simulink model "vblast_MMSE"  (Simulink 7.6)
settings: Solver=ode45  StartTime=0.0  StopTime=10.0  RelTol=1e-3
libraries: commchan3 x12, commdigbbndpm3 x2, dspindex x2, commrandsrc2 x1, commsink2 x1, dspinverses x1
settings Model: Creator=Administrator  LastModifiedBy=Administrator

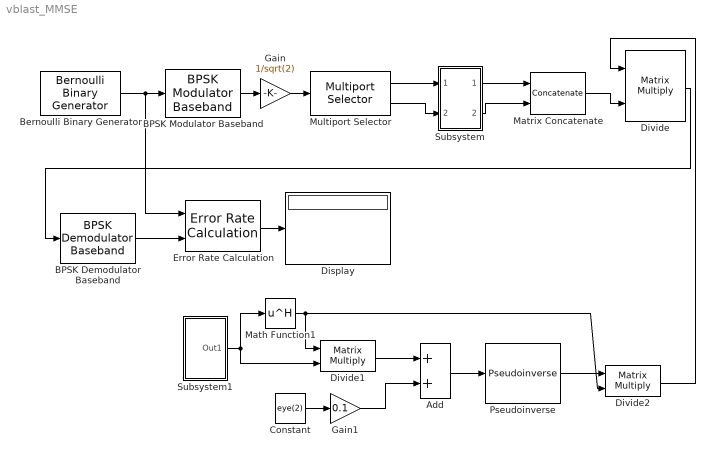
== system vblast_MMSE ==
  Add : Sum
  BPSK Demodulator Baseband : commdigbbndpm3/BPSK Demodulator Baseband  DialogController=commDDGCreate  DialogControllerArgs=DataTag0  Ph=0  DecType=Hard decision  VarSource=Dialog  Variance=1  outDtype=Inherit via internal rule  derotateFactorWordLen=16
  BPSK Modulator Baseband : commdigbbndpm3/BPSK Modulator Baseband  DialogController=commDDGCreate  DialogControllerArgs=DataTag1  SystemSampleTime=-1  Ph=0  outDtype=double  outWordLen=16  outUDDataType=sfix(16)  outFracLenMode=Best precision  outFracLen=15
  Bernoulli Binary Generator : commrandsrc2/Bernoulli Binary Generator  DialogController=commDDGCreate  DialogControllerArgs=DataTag2  SystemSampleTime=-1  P=0.5  seed=61  Ts=1e-6  frameBased=on  sampPerFrame=2  orient=off  outDataType=double
  Constant : Constant  Value=eye(2)
  Display : Display
  Divide : Product  Inputs=**  Multiplication=Matrix(*)
  Divide1 : Product  Inputs=**  Multiplication=Matrix(*)
  Divide2 : Product  Inputs=**  Multiplication=Matrix(*)
  Error Rate Calculation : commsink2/Error Rate Calculation  N=0  st_delay=0  cp_mode=Entire frame  subframe=[]  PMode=Port  WsName=ErrorVec  RsMode2=off  stop=off  numErr=100  maxBits=1e6
  Gain : Gain  Gain=1/sqrt(2)
  Gain1 : Gain  Gain=0.1
  Math Function1 : Math  Operator=hermitian  SaturateOnIntegerOverflow=on
  Matrix Concatenate : Concatenate  Mode=Multidimensional array
  Multiport Selector : dspindex/Multiport Selector  rowsOrCols=Rows  idxCellArray={ 1,2 }  idxErrMode=Clip Index
  Pseudoinverse : dspinverses/Pseudoinverse  wanterr=off
  Subsystem : Subsystem
  Subsystem1 : Subsystem
  wires:
  Bernoulli Binary Generator/1 -> BPSK Modulator Baseband/1, Error Rate Calculation/1
  BPSK Modulator Baseband/1 -> Gain/1
  Gain/1 -> Multiport Selector/1
  Subsystem/1(Out1) -> Matrix Concatenate/1
  Subsystem/2(Out2) -> Matrix Concatenate/2
  Multiport Selector/1 -> Subsystem/1(In1)
  Multiport Selector/2 -> Subsystem/2(In2)
  BPSK Demodulator Baseband/1 -> Error Rate Calculation/2
  Error Rate Calculation/1 -> Display/1
  Matrix Concatenate/1 -> Divide/2
  Divide/1 -> BPSK Demodulator Baseband/1
  Subsystem1/1(Out1) -> Math Function1/1, Divide1/2
  Math Function1/1 -> Divide1/1, Divide2/2
  Constant/1 -> Gain1/1
  Divide1/1 -> Add/1
  Gain1/1 -> Add/2
  Add/1 -> Pseudoinverse/1
  Pseudoinverse/1 -> Divide2/1
  Divide2/1 -> Divide/1

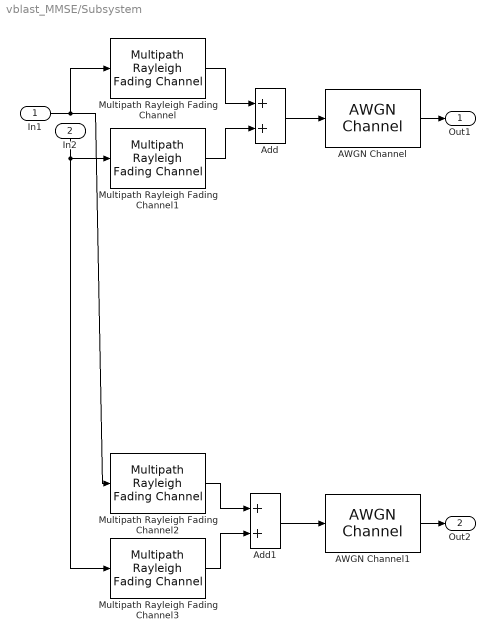
== system vblast_MMSE/Subsystem ==
  In1 : Inport
  In2 : Inport  Port=2
  AWGN Channel : commchan3/AWGN Channel  SystemSampleTime=-1  InputProcessing=Columns as channels (frame based)  seed=67  noiseMode="Signal to noise ratio  (SNR)"  EbNodB=10  EsNodB=10  SNRdB=10  bitsPerSym=1  Ps=1  Tsym=1  variance=1
  AWGN Channel1 : commchan3/AWGN Channel  SystemSampleTime=-1  InputProcessing=Columns as channels (frame based)  seed=671  noiseMode="Signal to noise ratio  (SNR)"  EbNodB=10  EsNodB=10  SNRdB=10  bitsPerSym=1  Ps=1  Tsym=1  variance=1
  Add : Sum
  Add1 : Sum
  Multipath Rayleigh Fading Channel : commchan3/Multipath Rayleigh Fading Channel  SystemSampleTime=-1  maxDopplerShift=40  spectrumType=Jakes  sigmaGaussian=1/sqrt(2)  coeffRounded=[1 -1.72 0.785]  freqMinMaxRJakes=[0 1]  freqMinMaxAJakes=[0 1]  sigmaGaussian1=1/sqrt(2)  sigmaGaussian2=1/sqrt(2)  centerFreqGaussian1=0.0  centerFreqGaussian2=0.0  gainGaussian1=0.5  gainGaussian2=0.5  coeffBell=9  dopplerSpectrum=doppler.jakes  pathDelays=0  avgPathGaindB=0  normalizePathGains=on  seed=73  enableProbe=0  openVisAtStart=off  outPathGains=off  outDelay=off
  Multipath Rayleigh Fading Channel1 : commchan3/Multipath Rayleigh Fading Channel  SystemSampleTime=-1  maxDopplerShift=40  spectrumType=Jakes  sigmaGaussian=1/sqrt(2)  coeffRounded=[1 -1.72 0.785]  freqMinMaxRJakes=[0 1]  freqMinMaxAJakes=[0 1]  sigmaGaussian1=1/sqrt(2)  sigmaGaussian2=1/sqrt(2)  centerFreqGaussian1=0.0  centerFreqGaussian2=0.0  gainGaussian1=0.5  gainGaussian2=0.5  coeffBell=9  dopplerSpectrum=doppler.jakes  pathDelays=0  avgPathGaindB=0  normalizePathGains=on  seed=731  enableProbe=0  openVisAtStart=off  outPathGains=off  outDelay=off
  Multipath Rayleigh Fading Channel2 : commchan3/Multipath Rayleigh Fading Channel  SystemSampleTime=-1  maxDopplerShift=40  spectrumType=Jakes  sigmaGaussian=1/sqrt(2)  coeffRounded=[1 -1.72 0.785]  freqMinMaxRJakes=[0 1]  freqMinMaxAJakes=[0 1]  sigmaGaussian1=1/sqrt(2)  sigmaGaussian2=1/sqrt(2)  centerFreqGaussian1=0.0  centerFreqGaussian2=0.0  gainGaussian1=0.5  gainGaussian2=0.5  coeffBell=9  dopplerSpectrum=doppler.jakes  pathDelays=0  avgPathGaindB=0  normalizePathGains=on  seed=7311  enableProbe=0  openVisAtStart=off  outPathGains=off  outDelay=off
  Multipath Rayleigh Fading Channel3 : commchan3/Multipath Rayleigh Fading Channel  SystemSampleTime=-1  maxDopplerShift=40  spectrumType=Jakes  sigmaGaussian=1/sqrt(2)  coeffRounded=[1 -1.72 0.785]  freqMinMaxRJakes=[0 1]  freqMinMaxAJakes=[0 1]  sigmaGaussian1=1/sqrt(2)  sigmaGaussian2=1/sqrt(2)  centerFreqGaussian1=0.0  centerFreqGaussian2=0.0  gainGaussian1=0.5  gainGaussian2=0.5  coeffBell=9  dopplerSpectrum=doppler.jakes  pathDelays=0  avgPathGaindB=0  normalizePathGains=on  seed=73111  enableProbe=0  openVisAtStart=off  outPathGains=off  outDelay=off
  Out1 : Outport
  Out2 : Outport  Port=2
  wires:
  In1/1 -> Multipath Rayleigh Fading Channel2/1, Multipath Rayleigh Fading Channel/1
  In2/1 -> Multipath Rayleigh Fading Channel3/1, Multipath Rayleigh Fading Channel1/1
  Multipath Rayleigh Fading Channel/1 -> Add/1
  Multipath Rayleigh Fading Channel1/1 -> Add/2
  Add/1 -> AWGN Channel/1
  Multipath Rayleigh Fading Channel2/1 -> Add1/1
  Multipath Rayleigh Fading Channel3/1 -> Add1/2
  Add1/1 -> AWGN Channel1/1
  AWGN Channel/1 -> Out1/1
  AWGN Channel1/1 -> Out2/1

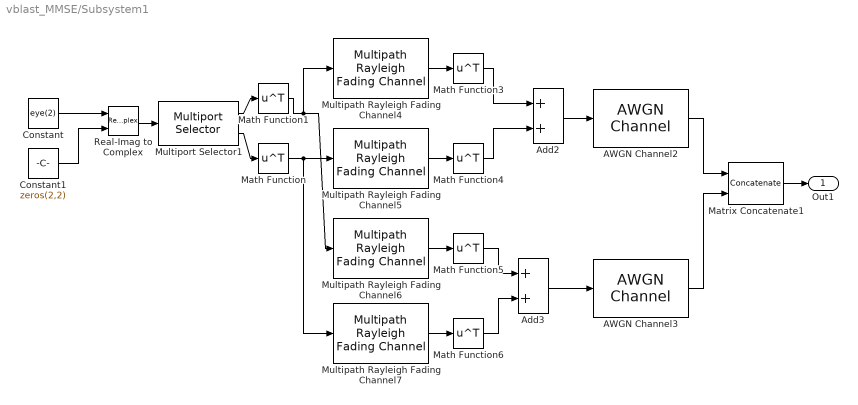
== system vblast_MMSE/Subsystem1 ==
  AWGN Channel2 : commchan3/AWGN Channel  SystemSampleTime=-1  InputProcessing=Columns as channels (frame based)  seed=67  noiseMode="Signal to noise ratio  (SNR)"  EbNodB=10  EsNodB=10  SNRdB=10  bitsPerSym=1  Ps=1  Tsym=1  variance=1
  AWGN Channel3 : commchan3/AWGN Channel  SystemSampleTime=-1  InputProcessing=Columns as channels (frame based)  seed=671  noiseMode="Signal to noise ratio  (SNR)"  EbNodB=10  EsNodB=10  SNRdB=10  bitsPerSym=1  Ps=1  Tsym=1  variance=1
  Add2 : Sum
  Add3 : Sum
  Constant : Constant  Value=eye(2)
  Constant1 : Constant  Value=zeros(2,2)
  Math Function{,1,3..6} (6 alike) : Math  Operator=transpose  SaturateOnIntegerOverflow=on
  Matrix Concatenate1 : Concatenate  Mode=Multidimensional array
  Multipath Rayleigh Fading Channel4 : commchan3/Multipath Rayleigh Fading Channel  SystemSampleTime=-1  maxDopplerShift=40  spectrumType=Jakes  sigmaGaussian=1/sqrt(2)  coeffRounded=[1 -1.72 0.785]  freqMinMaxRJakes=[0 1]  freqMinMaxAJakes=[0 1]  sigmaGaussian1=1/sqrt(2)  sigmaGaussian2=1/sqrt(2)  centerFreqGaussian1=0.0  centerFreqGaussian2=0.0  gainGaussian1=0.5  gainGaussian2=0.5  coeffBell=9  dopplerSpectrum=doppler.jakes  pathDelays=0  avgPathGaindB=0  normalizePathGains=on  seed=73  enableProbe=0  openVisAtStart=off  outPathGains=off  outDelay=off
  Multipath Rayleigh Fading Channel5 : commchan3/Multipath Rayleigh Fading Channel  SystemSampleTime=-1  maxDopplerShift=40  spectrumType=Jakes  sigmaGaussian=1/sqrt(2)  coeffRounded=[1 -1.72 0.785]  freqMinMaxRJakes=[0 1]  freqMinMaxAJakes=[0 1]  sigmaGaussian1=1/sqrt(2)  sigmaGaussian2=1/sqrt(2)  centerFreqGaussian1=0.0  centerFreqGaussian2=0.0  gainGaussian1=0.5  gainGaussian2=0.5  coeffBell=9  dopplerSpectrum=doppler.jakes  pathDelays=0  avgPathGaindB=0  normalizePathGains=on  seed=731  enableProbe=0  openVisAtStart=off  outPathGains=off  outDelay=off
  Multipath Rayleigh Fading Channel6 : commchan3/Multipath Rayleigh Fading Channel  SystemSampleTime=-1  maxDopplerShift=40  spectrumType=Jakes  sigmaGaussian=1/sqrt(2)  coeffRounded=[1 -1.72 0.785]  freqMinMaxRJakes=[0 1]  freqMinMaxAJakes=[0 1]  sigmaGaussian1=1/sqrt(2)  sigmaGaussian2=1/sqrt(2)  centerFreqGaussian1=0.0  centerFreqGaussian2=0.0  gainGaussian1=0.5  gainGaussian2=0.5  coeffBell=9  dopplerSpectrum=doppler.jakes  pathDelays=0  avgPathGaindB=0  normalizePathGains=on  seed=7311  enableProbe=0  openVisAtStart=off  outPathGains=off  outDelay=off
  Multipath Rayleigh Fading Channel7 : commchan3/Multipath Rayleigh Fading Channel  SystemSampleTime=-1  maxDopplerShift=40  spectrumType=Jakes  sigmaGaussian=1/sqrt(2)  coeffRounded=[1 -1.72 0.785]  freqMinMaxRJakes=[0 1]  freqMinMaxAJakes=[0 1]  sigmaGaussian1=1/sqrt(2)  sigmaGaussian2=1/sqrt(2)  centerFreqGaussian1=0.0  centerFreqGaussian2=0.0  gainGaussian1=0.5  gainGaussian2=0.5  coeffBell=9  dopplerSpectrum=doppler.jakes  pathDelays=0  avgPathGaindB=0  normalizePathGains=on  seed=73111  enableProbe=0  openVisAtStart=off  outPathGains=off  outDelay=off
  Multiport Selector1 : dspindex/Multiport Selector  rowsOrCols=Rows  idxCellArray={ 1,2 }  idxErrMode=Clip Index
  Real-Imag to Complex : RealImagToComplex
  Out1 : Outport
  wires:
  Multiport Selector1/1 -> Math Function1/1
  Multiport Selector1/2 -> Math Function/1
  Multipath Rayleigh Fading Channel4/1 -> Math Function3/1
  Multipath Rayleigh Fading Channel5/1 -> Math Function4/1
  Add2/1 -> AWGN Channel2/1
  Multipath Rayleigh Fading Channel6/1 -> Math Function5/1
  Multipath Rayleigh Fading Channel7/1 -> Math Function6/1
  Add3/1 -> AWGN Channel3/1
  Constant/1 -> Real-Imag to Complex/1
  Constant1/1 -> Real-Imag to Complex/2
  Real-Imag to Complex/1 -> Multiport Selector1/1
  Math Function1/1 -> Multipath Rayleigh Fading Channel6/1, Multipath Rayleigh Fading Channel4/1
  Math Function/1 -> Multipath Rayleigh Fading Channel7/1, Multipath Rayleigh Fading Channel5/1
  Math Function3/1 -> Add2/1
  Math Function4/1 -> Add2/2
  Math Function5/1 -> Add3/1
  Math Function6/1 -> Add3/2
  AWGN Channel2/1 -> Matrix Concatenate1/1
  AWGN Channel3/1 -> Matrix Concatenate1/2
  Matrix Concatenate1/1 -> Out1/1
